simulink model "DCE_motor6_V2"  (R2025a)
settings: Solver=ode4  StartTime=0.0  StopTime=1  FixedStep=5e-5  RelTol=1e-3
undefined symbols (not defined in the file or in its folder): powergui
libraries: spsControlledVoltageSourceLib x24, spsControlledCurrentSourceLib x24, spsVoltageMeasurementLib x24, slpidlib x24, spspowerguiLib x2, simulink x1
(part 1 of 5)
settings Model: Creator=One  LastModifiedBy=One

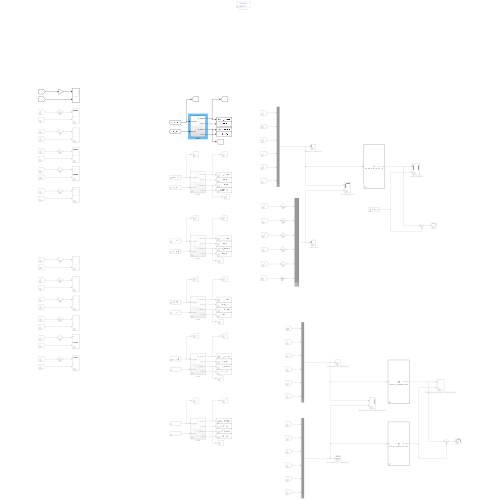
[thumbnail: Simulink's stored preview of the top-level diagram]
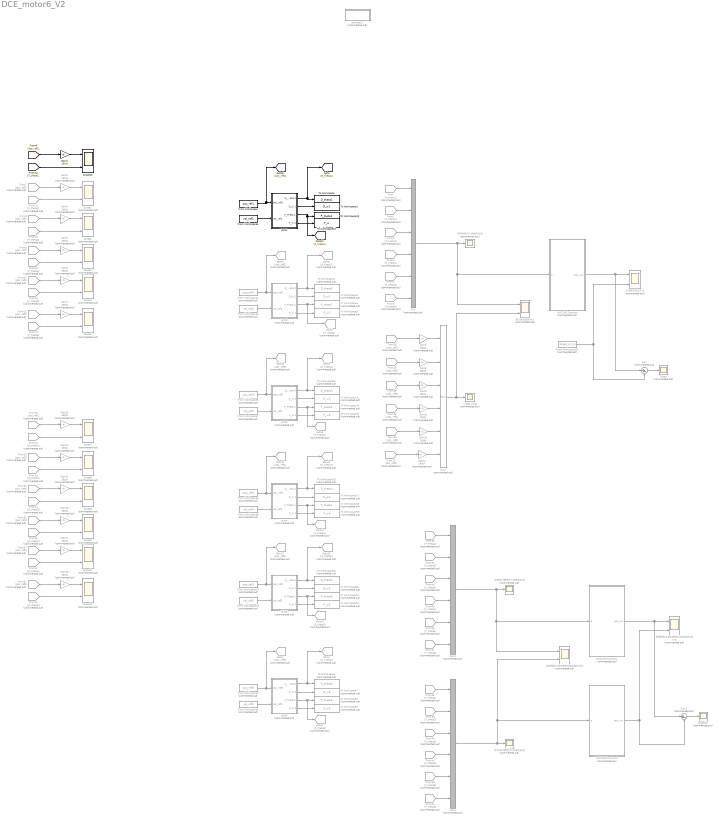
== system DCE_motor6_V2 ==
  From : From  Commented=on  GotoTag=P_theta1
  From Workspace : FromWorkspace  VariableName=pos_ref1
  From Workspace1 : FromWorkspace  VariableName=vel_ref1
  From Workspace10 : FromWorkspace  Commented=on  VariableName=pos_ref5
  From Workspace11 : FromWorkspace  Commented=on  VariableName=vel_ref5
  From Workspace12 : FromWorkspace  Commented=on  VariableName=target_xyz_ts
  From Workspace2 : FromWorkspace  Commented=on  VariableName=pos_ref2
  From Workspace3 : FromWorkspace  Commented=on  VariableName=vel_ref2
  From Workspace4 : FromWorkspace  Commented=on  VariableName=pos_ref6
  From Workspace5 : FromWorkspace  Commented=on  VariableName=vel_ref6
  From Workspace6 : FromWorkspace  Commented=on  VariableName=pos_ref3
  From Workspace7 : FromWorkspace  Commented=on  VariableName=vel_ref3
  From Workspace8 : FromWorkspace  Commented=on  VariableName=pos_ref4
  From Workspace9 : FromWorkspace  Commented=on  VariableName=vel_ref4
  From{1,13,37,39} (4 alike) : From  Commented=on  GotoTag=P_theta2
  From10 : From  Commented=on  GotoTag=pos_ref5
  From11 : From  Commented=on  GotoTag=pos_ref6
  From{2,14,40..41} (4 alike) : From  Commented=on  GotoTag=P_theta3
  From{3,15,42,45} (4 alike) : From  Commented=on  GotoTag=P_theta4
  From{4,16,43,46} (4 alike) : From  Commented=on  GotoTag=P_theta5
  From{5,17,44,47} (4 alike) : From  Commented=on  GotoTag=P_theta6
  From18 : From  Commented=on  GotoTag=pos_ref5
  From19 : From  Commented=on  GotoTag=pos_ref6
  From20 : From  Commented=on  GotoTag=pos_ref5
  From21 : From  Commented=on  GotoTag=pos_ref6
  From22 : From  Commented=on  GotoTag=D_theta1
  From23 : From  Commented=on  GotoTag=D_theta2
  From24 : From  Commented=on  GotoTag=D_theta3
  From25 : From  Commented=on  GotoTag=D_theta4
  From26 : From  Commented=on  GotoTag=pos_ref1
  From27 : From  Commented=on  GotoTag=pos_ref2
  From28 : From  Commented=on  GotoTag=pos_ref3
  From29 : From  Commented=on  GotoTag=pos_ref4
  From30 : From  Commented=on  GotoTag=D_theta5
  From31 : From  Commented=on  GotoTag=D_theta6
  From32 : From  Commented=on  GotoTag=pos_ref1
  From33 : From  Commented=on  GotoTag=pos_ref2
  From34 : From  Commented=on  GotoTag=pos_ref3
  From35 : From  Commented=on  GotoTag=pos_ref4
  From36 : From  Commented=on  GotoTag=P_theta1
  From38 : From  Commented=on  GotoTag=P_theta1
  From7 : From  Commented=on  GotoTag=pos_ref2
  From8 : From  Commented=on  GotoTag=pos_ref3
  From9 : From  Commented=on  GotoTag=pos_ref4
  Gain1 : Gain  Gain=180/pi
  Gain{2..18} (17 alike) : Gain  Commented=on  Gain=180/pi
  Goto1 : Goto  Commented=on  GotoTag=D_theta2
  Goto10 : Goto  Commented=on  GotoTag=pos_ref3
  Goto11 : Goto  Commented=on  GotoTag=D_theta4
  Goto13 : Goto  Commented=on  GotoTag=P_theta4
  Goto14 : Goto  Commented=on  GotoTag=pos_ref4
  Goto15 : Goto  Commented=on  GotoTag=D_theta5
  Goto16 : Goto  Commented=on  GotoTag=P_theta5
  Goto17 : Goto  Commented=on  GotoTag=pos_ref5
  Goto2 : Goto  Commented=on  GotoTag=P_theta2
  Goto3 : Goto  Commented=on  GotoTag=pos_ref2
  Goto4 : Goto  Commented=on  GotoTag=D_theta6
  Goto5 : Goto  Commented=on  GotoTag=P_theta6
  Goto7 : Goto  Commented=on  GotoTag=pos_ref6
  Goto8 : Goto  Commented=on  GotoTag=D_theta3
  Goto9 : Goto  Commented=on  GotoTag=P_theta3
  MATLAB Function : MATLAB Function  Commented=on  TreatAsAtomicUnit=on
  MATLAB Function1 : MATLAB Function  Commented=on  TreatAsAtomicUnit=on
  MATLAB Function2 : MATLAB Function  Commented=on  TreatAsAtomicUnit=on
  Mux{,1..3} (4 alike) : Mux  Commented=on  Inputs=6
  Scope : Scope  Commented=on
      settings: ActiveDisplayYMinimum=-0.000289462730006549  ActiveDisplayYMaximum=0.00023302341865344758  DataLoggingVariableName=ScopeData23
  Scope{1..9,11..12} (11 alike) : Scope  Commented=on  NumInputPorts=2
      Scope1 settings: ActiveDisplayYMinimum=-6.0139753089882335  ActiveDisplayYMaximum=54.125777780894119  DataLoggingVariableName=ScopeData10
      Scope11 settings: ActiveDisplayYMinimum=-48.669169301784144  ActiveDisplayYMaximum=5.4076854779760151
      Scope12 settings: ActiveDisplayYMinimum=-67.194027910067419  ActiveDisplayYMaximum=7.4660031011186
      Scope2 settings: ActiveDisplayYMinimum=-1.7922912289033655  ActiveDisplayYMaximum=12.011135261509935  DataLoggingVariableName=ScopeData16
      Scope3 settings: ActiveDisplayYMinimum=-8.3713341887105024  ActiveDisplayYMaximum=75.342007698394539  DataLoggingVariableName=ScopeData17
      Scope4 settings: ActiveDisplayYMinimum=-48.669169301784144  ActiveDisplayYMaximum=5.4076854779760151  DataLoggingVariableName=ScopeData18
      Scope5 settings: ActiveDisplayYMinimum=-67.194027910067419  ActiveDisplayYMaximum=7.4660031011186  DataLoggingVariableName=ScopeData19
      Scope6 settings: ActiveDisplayYMinimum=-6.0139753089882335  ActiveDisplayYMaximum=54.125777780894119  DataLoggingVariableName=ScopeData2
      Scope7 settings: ActiveDisplayYMinimum=43.128388243187558  ActiveDisplayYMaximum=44.899957966289  DataLoggingVariableName=ScopeData3
      Scope8 settings: ActiveDisplayYMinimum=-1.7922912289033655  ActiveDisplayYMaximum=12.011135261509935  DataLoggingVariableName=ScopeData4
      Scope9 settings: ActiveDisplayYMinimum=-8.3713341887105024  ActiveDisplayYMaximum=75.342007698394539  DataLoggingVariableName=ScopeData6
  Scope10 : Scope  NumInputPorts=2
      settings: ActiveDisplayYMinimum=-5.5836965217991938  ActiveDisplayYMaximum=7.5409112355633887  DataLoggingVariableName=ScopeData24
  Scope13 : Scope  Commented=on
      settings: ActiveDisplayYMinimum=-0.000289462730006549  ActiveDisplayYMaximum=0.00023302341865344758  DataLoggingVariableName=ScopeData7
  Sum : Sum  Commented=on  Inputs=|+-
  Sum1 : Sum  Commented=on  Inputs=|+-
  To Workspace : ToWorkspace  VariableName=D_theta1  SaveFormat=Timeseries  SampleTime=-1
  To Workspace1 : ToWorkspace  VariableName=D_w1  SaveFormat=Timeseries  SampleTime=-1
  To Workspace10 : ToWorkspace  Commented=on  VariableName=D_theta3  SaveFormat=Timeseries  SampleTime=-1
  To Workspace11 : ToWorkspace  Commented=on  VariableName=D_w3  SaveFormat=Timeseries  SampleTime=-1
  To Workspace12 : ToWorkspace  VariableName=P_theta1  SaveFormat=Timeseries  SampleTime=-1
  To Workspace13 : ToWorkspace  VariableName=P_w  SaveFormat=Timeseries  SampleTime=-1
  To Workspace14 : ToWorkspace  Commented=on  VariableName=P_theta3  SaveFormat=Timeseries  SampleTime=-1
  To Workspace15 : ToWorkspace  Commented=on  VariableName=P_w3  SaveFormat=Timeseries  SampleTime=-1
  To Workspace16 : ToWorkspace  Commented=on  VariableName=D_theta4  SaveFormat=Timeseries  SampleTime=-1
  To Workspace17 : ToWorkspace  Commented=on  VariableName=D_w4  SaveFormat=Timeseries  SampleTime=-1
  To Workspace18 : ToWorkspace  Commented=on  VariableName=P_theta4  SaveFormat=Timeseries  SampleTime=-1
  To Workspace19 : ToWorkspace  Commented=on  VariableName=P_w4  SaveFormat=Timeseries  SampleTime=-1
  To Workspace2 : ToWorkspace  Commented=on  VariableName=D_theta2  SaveFormat=Timeseries  SampleTime=-1
  To Workspace20 : ToWorkspace  Commented=on  VariableName=D_theta5  SaveFormat=Timeseries  SampleTime=-1
  To Workspace21 : ToWorkspace  Commented=on  VariableName=D_w5  SaveFormat=Timeseries  SampleTime=-1
  To Workspace22 : ToWorkspace  Commented=on  VariableName=P_theta5  SaveFormat=Timeseries  SampleTime=-1
  To Workspace23 : ToWorkspace  Commented=on  VariableName=P_w5  SaveFormat=Timeseries  SampleTime=-1
  To Workspace3 : ToWorkspace  Commented=on  VariableName=D_w2  SaveFormat=Timeseries  SampleTime=-1
  To Workspace4 : ToWorkspace  Commented=on  VariableName=P_theta2  SaveFormat=Timeseries  SampleTime=-1
  To Workspace5 : ToWorkspace  Commented=on  VariableName=P_w2  SaveFormat=Timeseries  SampleTime=-1
  To Workspace6 : ToWorkspace  Commented=on  VariableName=D_theta6  SaveFormat=Timeseries  SampleTime=-1
  To Workspace7 : ToWorkspace  Commented=on  VariableName=D_w6  SaveFormat=Timeseries  SampleTime=-1
  To Workspace8 : ToWorkspace  Commented=on  VariableName=P_theta6  SaveFormat=Timeseries  SampleTime=-1
  To Workspace9 : ToWorkspace  Commented=on  VariableName=P_w6  SaveFormat=Timeseries  SampleTime=-1
  joint1 : Subsystem
  joint2 : Subsystem  Commented=on
  joint3 : Subsystem  Commented=on
  joint4 : Subsystem  Commented=on
  joint5 : Subsystem  Commented=on
  joint6 : Subsystem  Commented=on
  powergui1 : Subsystem  Commented=on  AncestorBlock=spspowerguiLib/powergui  InitFcn=powergui( 'InitFcn_Callback' , gcb , 0 , [ ] );  mask(PSB option menu block){SimulationMode=Discrete, SampleTime=5e-5, frequency=60, Iterations=50, frequencyindice=0, Pbase=100e6, ErrMax=1e-4, UnitsV=kV, UnitsW=MW, buscounter=0, FunctionMessages=off, echomessages=off, EnableUseOfTLC=off, CurrentSourceSwitches=off, DisableSnubberDevices=off, DisableRonSwitches=off, DisableVfSwitches=off, DisplayEquations=off, AutomaticDiscreteSolvers=off, SolverType=Tustin/Backward Euler (TBE), Interpol=off, ExternalGateDelay=off, methode=off, Ts=0, x0status=blocks, SPID=off, SwTol=0, HookPort=off, NonlinearTolerance=1e-4, nMaxIteration=100, ContinueOnMaxIteration=off, RestoreLinks=warning, ResistiveCurrentMeasurement=off, Frange=[0:2:500], Ylog=off, Xlog=on, ShowGrid=off, save=off, variable=ZData, structure=0, ZoomFFT=on, StartTime=0.0, cycles=1, DisplayStyle=1, fundamental=60, FreqAxis=off, MaxFrequency=1000, frequencyindicesteady=1, RmsSteady=1, display=off}
      mask prompts: SimulationMode "Simulation type:"; SampleTime "Sample time (s):"; frequency "Frequency (Hz):"; Iterations "Max iterations"; frequencyindice "Frequency (Hz)"; Pbase "Base power (VA)"; ErrMax "PQ tolerance (pu)"; UnitsV "Voltage units"; UnitsW "Power units"; buscounter "Load flow bus counter"; FunctionMessages "Disable Specialized Power Systems warnings"; echomessages "Display Specialized Power Systems compilation messages"; EnableUseOfTLC "Use TLC file when in Accelerator Simulation Mode and for code generation"; CurrentSourceSwitches "Disable ideal switching"; DisableSnubberDevices "Disable snubbers in switching devices"; DisableRonSwitches "Disable Ron resistances in switching devices"; DisableVfSwitches "Disable forward voltages in switching devices"; DisplayEquations "Display circuit differential equations"; AutomaticDiscreteSolvers "Automatically handle Discrete solver and Advanced tab solver settings of blocks"; SolverType "Discrete solver"; Interpol "Interpolate switching events"; ExternalGateDelay "Use time-stamped gate signals"; methode "Store switching topologies"; Ts "Buffer size (MBytes):"; x0status "Start simulation with initial electrical states from:"; SPID "Use ideal switching devices"; SwTol "Switch tolerance"; HookPort "Allow multiple powergui blocks"; NonlinearTolerance "Solver tolerance"; nMaxIteration "Maximum number of iterations"; ContinueOnMaxIteration "Continue Simulation if maximum number of iterations is reached"; RestoreLinks "Restore disabled links of Simscape Power Systems ST blocks:"; ResistiveCurrentMeasurement "Use non ideal current measurement blocks (1e-4Ohm internal resistance)"; Frange "Frequency Range"; Ylog "Log impedance"; Xlog "log Frequency"; ShowGrid "grid"; save "Save Data To Workspace"; variable "Variable Name"; structure "Structure Name (PSBFFTSCOPE)"; ZoomFFT "ZoomFFT (PSBFFTSCOPE)"; StartTime "Start Time (PSBFFTSCOPE)"; cycles "Cycles (PSBFFTSCOPE)"; DisplayStyle "Display style (PSBFFTSCOPE)"; fundamental "Fundamental (PSBFFTSCOPE)"; FreqAxis "Frequency Axis (PSBFFTSCOPE)"; MaxFrequency "Max Frequency (PSBFFTSCOPE)"; frequencyindicesteady "Frequency indice (STEADYSTATE)"; RmsSteady "RMS display (STEADYSTATE)"; display "Display Results"
      mask help: Set simulation type, simulation parameters, and preferences.
      mask init:
      | dispMessage = '';
      | dispMessage = powergui('MaskInitialization',gcb,SimulationMode,SampleTime);
      settings: PreSaveFcn=powergui( 'PreSaveFcn_Callback' , gcb , [ ] , [ ] );  OpenFcn=sps_rtmsupport('OpenFcn',gcbh)
      mask Help: helpview(psbhelp)
      mask TypeOptions SimulationMode: Continuous | Discrete | Phasor | Discrete phasor
      mask Callback SimulationMode: powergui('SimulationType',[],[],gcb);
      mask TypeOptions UnitsV: V | kV
      mask TypeOptions UnitsW: W | kW | MW
      mask Callback CurrentSourceSwitches: powergui('SimulationType',[],[],gcb);
      mask Callback AutomaticDiscreteSolvers: powergui('SimulationType',[],[],gcb);
      mask TypeOptions SolverType: Tustin/Backward Euler (TBE) | Tustin | Backward Euler
      mask Callback SolverType: powergui('SimulationType',[],[],gcb);
      mask Callback Interpol: powergui('SimulationType',[],[],gcb);
      mask Callback ExternalGateDelay: powergui('SimulationType',[],[],gcb);
      mask Callback methode: powergui('SimulationType',[],[],gcb);
      mask TypeOptions x0status: blocks | steady | zero
      mask TypeOptions RestoreLinks: yes | warning | no
      mask Callback display: sps_rtmsupport('parametereditingmodes',gcbh) % Will be executed last in parameter callbacks to ensure mask enable consistency
      mask DialogControl SolverTab Prompt: Solver
      mask DialogControl AutoSolverNote Prompt: The Simulation type parameter is governed by Simulink. To access the Powergui solver settings, unselect auto (Automatic solver selection) solver in the Simulink solver options.
      mask DialogControl Apps Prompt: Apps
      mask DialogControl StateAnalyzer Prompt: Measurements and States Analyzer
      mask DialogControl StateAnalyzer Callback: powerStates(bdroot(gcb))
      mask DialogControl LineParameterCalculator Prompt: Line Parameter Calculator
      mask DialogControl LineParameterCalculator Callback:
      | close_system(gcb)
      | powerLineParameters
      mask DialogControl CableParameterCalculator Prompt: Cable Parameter Calculator
      mask DialogControl CableParameterCalculator Callback:
      | close_system(gcb)
      | powerCableParameters
      mask DialogControl LineDecoupler Prompt: Line Decoupler
      mask DialogControl LineDecoupler Tooltip: Click to replace selected Distributed Parameters Line blocks with Decoupling Line blocks
      mask DialogControl LineDecoupler Callback:
      | close_system(gcb);
      | DecouplingLineReplace(gcs)
      mask DialogControl LoadFlowAnalyzer Prompt: Load Flow Analyzer
      mask DialogControl LoadFlowAnalyzer Callback:
      | close_system(gcb)
      | powerLoadFlow
      mask DialogControl LoadFlowParameters Prompt: Load Flow Parameters
      mask DialogControl ImpedanceCalculator Prompt: Impedance Calculator
      mask DialogControl ImpedanceCalculator Callback:
      | close_system(gcb);
      | powerImpedance(bdroot(gcs));
      mask DialogControl FFTAnalyzer Prompt: FFT Analyzer
      mask DialogControl FFTAnalyzer Callback:
      | close_system(gcb)
      | power_fftscope(bdroot(gcb),gcb)
      mask DialogControl LinearSystemAnalyzer Prompt: Linear System Analyzer
      mask DialogControl LinearSystemAnalyzer Callback:
      | close_system(gcb)
      | power_ltiview(bdroot(gcb))
      mask DialogControl HysteresisDesigner Prompt: Hysteresis Designer
      mask DialogControl HysteresisDesigner Callback:
      | close_system(gcb)
      | powerHysteresis('hysteresis.mat')
      mask DialogControl BlockCustomizer Prompt: Block Customizer
      mask DialogControl BlockCustomizer Callback:
      | close_system(gcb);
      | power_customize;
      mask DialogControl ReportGenerator Prompt: Report Generator
      mask DialogControl ReportGenerator Callback:
      | close_system(gcb)
      | power_report(bdroot(gcb))
      mask DialogControl obsolete Prompt: ...
      mask DialogControl MachineInitialization Prompt: Machine Initialization
      mask DialogControl MachineInitialization Callback:
      | close_system(gcb)
      | powericon('machineInitTool',bdroot(gcb),gcb)
      mask DialogControl Preferences Prompt: Preferences
      mask DialogControl Solver Prompt: Solver
      mask DialogControl SolverDetails Prompt: Solver details for nonlinear elements
      mask Display: color('blue'),disp(dispMessage)
  六条输入轨迹 : Scope  Commented=on
      settings: DataLoggingVariableName=ScopeData20
  实物电机模型的六条输出轨迹 : Scope  Commented=on
      settings: ActiveDisplayYMinimum=-75.563478283435458  ActiveDisplayYMaximum=82.802808576726292  DataLoggingVariableName=ScopeData9
  实物电机的六条输出轨迹 : Scope  Commented=on
      settings: ActiveDisplayYMinimum=-75.563478283435458  ActiveDisplayYMaximum=82.802808576726292  DataLoggingVariableName=ScopeData15
  尖端电机轨迹XYZ : Scope  Commented=on  NumInputPorts=2
      settings: ActiveDisplayYMinimum=-0.074441825005112566  ActiveDisplayYMaximum=0.66483489550037078  DataLoggingVariableName=ScopeData22
  数字电机模型的六条输出轨迹 : Scope  Commented=on
      settings: DataLoggingVariableName=ScopeData8
  物理模型与数字模型的尖端电机轨迹XYZ : Scope  Commented=on  NumInputPorts=2
      settings: ActiveDisplayYMinimum=-0.061507125001366951  ActiveDisplayYMaximum=0.37025412500015187  DataLoggingVariableName=ScopeData11
  物理模型与数字模型的输出曲线对比 : Scope  Commented=on  NumInputPorts=2
      settings: ActiveDisplayYMinimum=-75.563478283435458  ActiveDisplayYMaximum=82.802808576726292  DataLoggingVariableName=ScopeData12
  输入输出曲线对比 : Scope  Commented=on  NumInputPorts=2
      settings: ActiveDisplayYMinimum=-75.563478283435458  ActiveDisplayYMaximum=82.802808576726292  DataLoggingVariableName=ScopeData21
  wires:
  From/1 -> Mux/1
  From1/1 -> Mux/2
  From2/1 -> Mux/3
  From3/1 -> Mux/4
  From4/1 -> Mux/5
  From5/1 -> Mux/6
  Mux/1 -> MATLAB Function/1(q), 输入输出曲线对比/1, 实物电机的六条输出轨迹/1
  [pos_ref1] -> Gain1/1
  From7/1 -> Gain2/1
  From8/1 -> Gain4/1
  From9/1 -> Gain5/1
  From10/1 -> Gain6/1
  From11/1 -> Gain7/1
  Gain1/1 -> Scope10/1
  Gain2/1 -> Scope1/1
  Gain4/1 -> Scope2/1
  Gain5/1 -> Scope3/1
  Gain6/1 -> Scope4/1
  Gain7/1 -> Scope5/1
  [P_theta1] -> Scope10/2
  From13/1 -> Scope1/2
  From14/1 -> Scope2/2
  From15/1 -> Scope3/2
  From16/1 -> Scope4/2
  From17/1 -> Scope5/2
  From26/1 -> Gain3/1
  From27/1 -> Gain8/1
  Gain3/1 -> Mux1/1
  From28/1 -> Gain9/1
  From29/1 -> Gain10/1
  Gain11/1 -> Mux1/5
  From19/1 -> Gain12/1
  Gain10/1 -> Mux1/4
  Gain12/1 -> Mux1/6
  Gain8/1 -> Mux1/2
  From18/1 -> Gain11/1
  Gain9/1 -> Mux1/3
  Mux1/1 -> 输入输出曲线对比/2, 六条输入轨迹/1
  MATLAB Function/1(pos_xyz) -> Sum/1, 尖端电机轨迹XYZ/1
  From Workspace12/1 -> Sum/2, 尖端电机轨迹XYZ/2
  Sum/1 -> Scope/1
  From Workspace/1 -> [pos_ref1], joint1/1(pos_ref1)
  From Workspace1/1 -> joint1/2(vel_ref1)
  joint1/1(D_Theta 1) -> To Workspace/1, [D_theta1]
  joint1/2(D_w 1) -> To Workspace1/1
  joint1/3(P_Theta 1) -> [P_theta1], To Workspace12/1
  joint1/4(P_w 1) -> To Workspace13/1
  From Workspace3/1 -> joint2/2(vel_ref2)
  joint2/2(D_w 2) -> To Workspace3/1
  joint2/3(P_Theta 2) -> Goto2/1, To Workspace4/1
  joint2/4(P_w 2) -> To Workspace5/1
  joint2/1(D_Theta 2) -> To Workspace2/1, Goto1/1
  From Workspace2/1 -> Goto3/1, joint2/1(pos_ref2)
  From Workspace7/1 -> joint3/2(vel_ref3)
  joint3/2(D_w 3) -> To Workspace11/1
  joint3/3(P_Theta 3) -> Goto9/1, To Workspace14/1
  joint3/4(P_w 3) -> To Workspace15/1
  joint3/1(D_Theta 3) -> To Workspace10/1, Goto8/1
  From Workspace6/1 -> Goto10/1, joint3/1(pos_ref3)
  From Workspace9/1 -> joint4/2(vel_ref4)
  joint4/2(D_w 4) -> To Workspace17/1
  joint4/3(P_Theta 4) -> Goto13/1, To Workspace18/1
  joint4/4(P_w 4) -> To Workspace19/1
  joint4/1(D_Theta 4) -> To Workspace16/1, Goto11/1
  From Workspace8/1 -> Goto14/1, joint4/1(pos_ref4)
  From Workspace11/1 -> joint5/2(vel_ref5)
  joint5/2(D_w 5) -> To Workspace21/1
  joint5/3(P_Theta 5) -> Goto16/1, To Workspace22/1
  joint5/4(P_w 5) -> To Workspace23/1
  joint5/1(D_Theta 5) -> To Workspace20/1, Goto15/1
  From Workspace10/1 -> Goto17/1, joint5/1(pos_ref5)
  joint6/1(D_Theta 6) -> To Workspace6/1, Goto4/1
  joint6/2(D_w 6) -> To Workspace7/1
  joint6/4(P_w 6) -> To Workspace9/1
  joint6/3(P_Theta 6) -> Goto5/1, To Workspace8/1
  From Workspace5/1 -> joint6/2(vel_ref6)
  From Workspace4/1 -> Goto7/1, joint6/1(pos_ref6)
  From30/1 -> Scope11/2
  From25/1 -> Scope9/2
  From22/1 -> Scope7/2
  Gain17/1 -> Scope11/1
  From23/1 -> Scope6/2
  From24/1 -> Scope8/2
  Gain15/1 -> Scope8/1
  From31/1 -> Scope12/2
  Gain14/1 -> Scope6/1
  From33/1 -> Gain14/1
  Gain16/1 -> Scope9/1
  From32/1 -> Gain13/1
  Gain18/1 -> Scope12/1
  From20/1 -> Gain17/1
  From21/1 -> Gain18/1
  From34/1 -> Gain15/1
  From35/1 -> Gain16/1
  Gain13/1 -> Scope7/1
  From37/1 -> Mux2/2
  From47/1 -> Mux2/6
  MATLAB Function1/1(pos_xyz) -> Sum1/1, 物理模型与数字模型的尖端电机轨迹XYZ/1
  From46/1 -> Mux2/5
  From36/1 -> Mux2/1
  Sum1/1 -> Scope13/1
  From40/1 -> Mux2/3
  From45/1 -> Mux2/4
  Mux2/1 -> MATLAB Function1/1(q), 物理模型与数字模型的输出曲线对比/1, 实物电机模型的六条输出轨迹/1
  Mux3/1 -> 物理模型与数字模型的输出曲线对比/2, MATLAB Function2/1(q), 数字电机模型的六条输出轨迹/1
  From42/1 -> Mux3/4
  From41/1 -> Mux3/3
  From38/1 -> Mux3/1
  From44/1 -> Mux3/6
  From43/1 -> Mux3/5
  From39/1 -> Mux3/2
  MATLAB Function2/1(pos_xyz) -> Sum1/2, 物理模型与数字模型的尖端电机轨迹XYZ/2

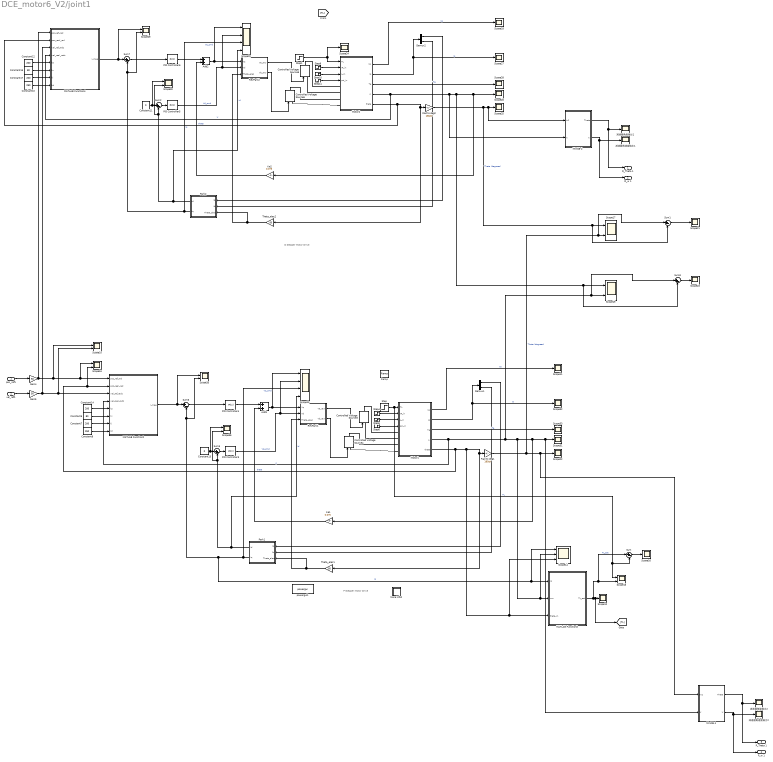
== system DCE_motor6_V2/joint1 ==
  note: D Stepper Motor Drive
  note: P Stepper Motor Drive
  pos_ref1 : Inport
  vel_ref1 : Inport  Port=2
  Add1 : Sum
  Add2 : Sum
  Constant10 : Constant  Value=250
  Constant11 : Constant  Value=0
  Constant{7,12,14,17} (4 alike) : Constant  Value=200
  Constant13 : Constant  Value=0
  Constant15 : Constant  Value=80
  Constant6 : Constant  Value=80
  Constant8 : Constant  Value=250
  Controlled Voltage Source{3..6} (4 alike) : spsControlledVoltageSourceLib/Controlled Voltage Source  Initialize=on  Source_Type=AC  Amplitude=0  Phase=0  Frequency=0  Measurements=None
  Demux1 : Demux  Outputs=2
  Demux2 : Demux  Outputs=2
  Gain4 : Gain  Gain=50
  Gain5 : Gain  Gain=50
  Ke1 : Gain  Gain=0.075
  Ke2 : Gain  Gain=0.075
  MATLAB Function2 : MATLAB Function  TreatAsAtomicUnit=on
  MATLAB Function3 : MATLAB Function  TreatAsAtomicUnit=on
  MATLAB Function4 : MATLAB Function  TreatAsAtomicUnit=on
  Mini08-1 : Subsystem
  Mini08-2 : Subsystem
  More Info2 : Subsystem
      settings: OpenFcn="showExample(\"simscapeelectricalsps/StepperMotorExample\")"
      mask Display: disp('?')
  Motor1 : Subsystem
  Motor2 : Subsystem
  PID Controller{3..6} (4 alike) : slpidlib/PID Controller  Controller=PI  Form=Parallel  TimeDomain=Discrete-time  UseExternalTs=off  SampleTime=5e-5  IntegratorMethod=Forward Euler  FilterMethod=Forward Euler  ControllerParametersSource=internal  P=5  I=4000  UseKiTs=off  D=0  UseExternalDerivativeSource=off  N=100  UseFilter=on  TunerSelectOption=Transfer Function Based (PID Tuner App)  InitialConditionSource=internal  InitialConditionForIntegrator=0  InitialConditionForFilter=0  DifferentiatorICPrevScaledInput=0  ExternalReset=none  TrackingMode=off  Kt=1  LimitOutput=on  SatLimitsSource=internal  UpperSaturationLimit=24  LowerSaturationLimit=-24  LinearizeAsGain=on  AntiWindupMode=clamping  Kb=1  LimitIntegrator=on  UpperIntegratorSaturationLimit=24  LowerIntegratorSaturationLimit=-24  POutMin=[]  POutMax=[]  IOutMin=[]  IOutMax=[]  DOutMin=[]  DOutMax=[]  NOutMin=[]  NOutMax=[]  SumOutMin=[]  SumOutMax=[]  SaturationOutMin=[]  SaturationOutMax=[]  PParamMin=[]  PParamMax=[]  IParamMin=[]  IParamMax=[]  DParamMin=[]  DParamMax=[]  NParamMin=[]  NParamMax=[]  KbParamMin=[]  KbParamMax=[]  KtParamMin=[]  KtParamMax=[]  KbOutMin=[]  KbOutMax=[]  KtOutMin=[]  KtOutMax=[]  IntegratorOutMin=[]  IntegratorOutMax=[]  FilterOutMin=[]  FilterOutMax=[]  SumI1OutMin=[]  SumI1OutMax=[]  SumI2OutMin=[]  SumI2OutMax=[]  SumI3OutMin=[]  SumI3OutMax=[]  SumI4OutMin=[]  SumI4OutMax=[]  SumDOutMin=[]  SumDOutMax=[]  DifferentiatorOutMin=[]  DifferentiatorOutMax=[]  FilterDiffOutCoefMin=[]  FilterDiffOutCoefMax=[]  ReciprocalOutMin=[]  ReciprocalOutMax=[]  SumDenOutMin=[]  SumDenOutMax=[]  SumNumOutMin=[]  SumNumOutMax=[]  DivideOutMin=[]  DivideOutMax=[]  UdiffTsProdOutMin=[]  UdiffTsProdOutMax=[]  NTsProdOutMin=[]  NTsProdOutMax=[]  UintegralTsProdOutMin=[]  UintegralTsProdOutMax=[]  UngainTsProdOutMin=[]  UngainTsProdOutMax=[]  ClampingZeroOutDataTypeStr=Inherit: Inherit via back propagation  ClampingZeroOutMin=[]  ClampingZeroOutMax=[]  FilterDenConstantOutDataTypeStr=Inherit: Inherit via back propagation  FilterDenConstantOutMin=[]  FilterDenConstantOutMax=[]  PCopyOutDataTypeStr=Inherit: Inherit via back propagation  PCopyOutMin=[]  PCopyOutMax=[]  NCopyOutDataTypeStr=Inherit: Inherit via back propagation  NCopyOutMin=[]  NCopyOutMax=[]  IntegratorContinuousStateAttributes=''  IntegratorStateMustResolveToSignalObject=off  IntegratorRTWStateStorageClass=Auto  FilterContinuousStateAttributes=''  FilterStateMustResolveToSignalObject=off  FilterRTWStateStorageClass=Auto  ParallelPVariant=InternalParameters  IdealPVariant=Disabled  IVariant=InternalParameters  DVariant=Disabled  IntegratorVariant=Discrete  SatVariant=Enabled  AWVariant=DiscClampingParallel  PCopyVariant=Disabled  TRVariant=Disabled  FdbkBlocksVariant=Forward  IdealPFdbkVariant=Disabled  SatFdbkVariant=Disabled  DerivativeFilterVariant=Disabled  NVariant=Disabled  NCopyVariant=Disabled_SignalSpec  FilterICVariant=Disabled  IntegratorICVariant=InternalICs  ExternalResetVariant=Disabled  TRSumVariant=Passthrough  SumFdbkVariant=Disabled  SumVariant=Sum_PI  TsampFilterVariant=InternalTs  TsampNgainVariant=Passthrough  TsampIntegralVariant=Disabled_SignalSpec  ExternalSaturationOutDataTypeStr=Inherit: Same as second input  DerivativeSourceVariant=Disabled  PreIntVariant=InternalPreInt
  Park1 : MATLAB Function  TreatAsAtomicUnit=on
  Park2 : MATLAB Function  TreatAsAtomicUnit=on
  Rad to deg1 : Gain  Gain=180/pi
  Rad to deg2 : Gain  Gain=180/pi
  Ramp : simulink/Sources/Ramp  slope=0.006  start=0  InitialOutput=0.01
  RevPark1 : MATLAB Function  TreatAsAtomicUnit=on
  RevPark2 : MATLAB Function  TreatAsAtomicUnit=on
  Scope{10,15,17,19,29..30,34..36} (9 alike) : Scope  NumInputPorts=2
      Scope10 settings: ActiveDisplayYMinimum=-5.2481835137744008  ActiveDisplayYMaximum=47.233651623969614  DataLoggingVariableName=ScopeData27
      Scope15 settings: ActiveDisplayYMinimum=0.00625  ActiveDisplayYMaximum=0.04375  DataLoggingVariableName=ScopeData34
      Scope17 settings: ActiveDisplayYMinimum=-287.89976310434338  ActiveDisplayYMaximum=575.16137858375225  DataLoggingVariableName=ScopeData36
      Scope19 settings: ActiveDisplayYMinimum=-24.982969715205265  ActiveDisplayYMaximum=69.499857868635672  DataLoggingVariableName=ScopeData38
      Scope29 settings: ActiveDisplayYMinimum=-0.018504547079538081  ActiveDisplayYMaximum=0.49853620070628168  DataLoggingVariableName=ScopeData28
      Scope30 settings: ActiveDisplayYMinimum=-0.068250226127922337  ActiveDisplayYMaximum=0.064256506451961737  DataLoggingVariableName=ScopeData29
      Scope34 settings: ActiveDisplayYMinimum=37.665150555747651  ActiveDisplayYMaximum=39.407336225091846  DataLoggingVariableName=ScopeData49
      Scope35 settings: ActiveDisplayYMinimum=-0.018504547079538081  ActiveDisplayYMaximum=0.49853620070628168  DataLoggingVariableName=ScopeData50
      Scope36 settings: ActiveDisplayYMinimum=-0.068250226127922337  ActiveDisplayYMaximum=0.064256506451961737  DataLoggingVariableName=ScopeData51
  Scope{11..12,16,18,21..28,31..33} (15 alike) : Scope
      Scope11 settings: ActiveDisplayYMinimum=-19.096901402816375  ActiveDisplayYMaximum=19.120590576315788  DataLoggingVariableName=ScopeData30
      Scope12 settings: ActiveDisplayYMinimum=-0.005028035303192257  ActiveDisplayYMaximum=0.045252317728730319  DataLoggingVariableName=ScopeData31
      Scope16 settings: ActiveDisplayYMinimum=-0.00045623090907525666  ActiveDisplayYMaximum=0.00044225246132360179  DataLoggingVariableName=ScopeData35
      Scope18 settings: ActiveDisplayYMinimum=-19.096901402816375  ActiveDisplayYMaximum=19.120590576315788  DataLoggingVariableName=ScopeData37
      Scope21 settings: ActiveDisplayYMinimum=-6.1502055823969322  ActiveDisplayYMaximum=1.5579460890257923  DataLoggingVariableName=ScopeData40
      Scope22 settings: ActiveDisplayYMinimum=-1073.0161987450256  ActiveDisplayYMaximum=478.45817124156184  DataLoggingVariableName=ScopeData41
      Scope23 settings: ActiveDisplayYMinimum=-6.5852940186487112  ActiveDisplayYMaximum=6.2413973243820795  DataLoggingVariableName=ScopeData42
      Scope24 settings: ActiveDisplayYMinimum=-0.019291388561127311  ActiveDisplayYMaximum=0.055061528118044607  DataLoggingVariableName=ScopeData43
      Scope25 settings: ActiveDisplayYMinimum=-101.39982984513261  ActiveDisplayYMaximum=451.43127016035271  DataLoggingVariableName=ScopeData44
      Scope26 settings: ActiveDisplayYMinimum=-452.6835395386438  ActiveDisplayYMaximum=318.93705127381384  DataLoggingVariableName=ScopeData45
      Scope27 settings: ActiveDisplayYMinimum=-0.40449771436693455  ActiveDisplayYMaximum=0.64067173662257559  DataLoggingVariableName=ScopeData25
      Scope28 settings: ActiveDisplayYMinimum=-0.046646220623980633  ActiveDisplayYMaximum=0.10063848186154864  DataLoggingVariableName=ScopeData26
      Scope31 settings: ActiveDisplayYMinimum=-108.68072883446378  ActiveDisplayYMaximum=111.31923817185427  DataLoggingVariableName=ScopeData46
      Scope32 settings: ActiveDisplayYMinimum=-0.40449771436693455  ActiveDisplayYMaximum=0.64067173662257559  DataLoggingVariableName=ScopeData47
      Scope33 settings: ActiveDisplayYMinimum=-0.046646220623980633  ActiveDisplayYMaximum=0.10063848186154864  DataLoggingVariableName=ScopeData48
  Scope13 : Scope  NumInputPorts=4
      settings: ActiveDisplayYMinimum=-0.68813129304418319  ActiveDisplayYMaximum=6.2555990509558841  DataLoggingVariableName=ScopeData32
  Scope14 : Scope  NumInputPorts=3
      settings: ActiveDisplayYMinimum=-0.052783691584462819  ActiveDisplayYMaximum=0.4750532242601655  DataLoggingVariableName=ScopeData33
  Scope20 : Scope  NumInputPorts=4
      settings: ActiveDisplayYMinimum=-0.68813129304418319  ActiveDisplayYMaximum=6.2555990509558841  DataLoggingVariableName=ScopeData39
  Step : Step  Time=0.5  Before=0.005  After=0.04  SampleTime=0
  Step1 : Step  Time=0  Before=0.005  After=0.005  SampleTime=0
  Step10 : Step  Time=0  Before=0.00544  After=0.00544  SampleTime=0
  Step11 : Step  Time=0  Before=0.0015  After=0.0015  SampleTime=0
  Step4 : Step  Time=0  Before=4.85  After=4.85  SampleTime=0
  Step5 : Step  Time=0  Before=0.00544  After=0.00544  SampleTime=0
  Step6 : Step  Time=0  Before=0.0015  After=0.0015  SampleTime=0
  Step9 : Step  Time=0  Before=4.85  After=4.85  SampleTime=0
  Sum{,1..2,5..8} (7 alike) : Sum  Inputs=|+-
  Theta_elec1 : Gain  Gain=50
  Theta_elec2 : Gain  Gain=50
  powergui1 : spspowerguiLib/powergui  SimulationMode=Discrete  SampleTime=5e-5  frequency=60  Iterations=50  frequencyindice=0  Pbase=100e6  ErrMax=1e-4  UnitsV=kV  UnitsW=MW  buscounter=0  FunctionMessages=off  echomessages=off  EnableUseOfTLC=off  CurrentSourceSwitches=off  DisableSnubberDevices=off  DisableRonSwitches=off  DisableVfSwitches=off  DisplayEquations=off  AutomaticDiscreteSolvers=off  SolverType=Tustin/Backward Euler (TBE)  Interpol=off  ExternalGateDelay=off  methode=off  Ts=0  x0status=blocks  SPID=off  SwTol=0  HookPort=off  NonlinearTolerance=1e-4  nMaxIteration=100  ContinueOnMaxIteration=off  RestoreLinks=warning  ResistiveCurrentMeasurement=off  Frange=[0:2:500]  Ylog=off  Xlog=on  ShowGrid=off  save=off  variable=ZData  structure=0  ZoomFFT=on  StartTime=0.0  cycles=1  DisplayStyle=1  fundamental=60  FreqAxis=off  MaxFrequency=1000  frequencyindicesteady=1  RmsSteady=1  display=off
  减速器角度输出1 : Scope
      settings: ActiveDisplayYMinimum=-3.2575204385667078  ActiveDisplayYMaximum=25.318176358378867  DataLoggingVariableName=ScopeData53
  减速器角度输出2 : Scope
      settings: ActiveDisplayYMinimum=-3.2575204385667078  ActiveDisplayYMaximum=25.318176358378867  DataLoggingVariableName=ScopeData56
  减速器角速度输出1 : Scope
      settings: ActiveDisplayYMinimum=-0.049701649268213327  ActiveDisplayYMaximum=0.44324985732957672  DataLoggingVariableName=ScopeData54
  减速器角速度输出2 : Scope
      settings: ActiveDisplayYMinimum=-0.049701649268213327  ActiveDisplayYMaximum=0.44324985732957672  DataLoggingVariableName=ScopeData57
  D_Theta 1 : Outport
  D_w 1 : Outport  Port=2
  P_Theta 1 : Outport  Port=3
  P_w 1 : Outport  Port=4
  wires:
  Sum8/1 -> Scope23/1
  Sum1/1 -> Scope21/1
  Motor2/1(Vp) -> Scope18/1  "Vp"
  Motor2/2(Ip) -> Demux2/1, Scope27/1  "Ip"
  Park2/2(Iq) -> Scope20/3, Scope29/2, Sum7/2  "Iq"
  Park2/1(Id) -> Scope20/4, Scope30/2, Sum2/2  "Id"
  Constant11/1 -> Scope30/1, Sum2/1
  PID Controller6/1 -> Add2/1
  MATLAB Function4/1(I_mag) -> Scope29/1, Sum7/1
  Demux2/1 -> Park2/1(Ia)
  Sum7/1 -> PID Controller6/1
  Motor2/5(theta) -> MATLAB Function4/2(pos_real_rad), Rad to deg2/1, Theta_elec2/1  "theta"
  Constant12/1 -> MATLAB Function4/5(kp)
  Sum2/1 -> PID Controller5/1
  Step10/1 -> Motor2/3(L_in)
  Ke2/1 -> Add2/2
  Motor2/3(Te) -> Scope28/1  "Te"
  RevPark2/2(Vb_raw) -> Controlled Voltage Source6/1
  Step11/1 -> Motor2/4(psi_in)
  Theta_elec2/1 -> RevPark2/3(Theta_elec), Park2/3(Theta_elec)
  Constant17/1 -> MATLAB Function4/7(ki)
  Add2/1 -> Scope20/1, RevPark2/1(Vq)  "Vq_cmd"
  PID Controller5/1 -> Scope20/2, RevPark2/2(Vd)  "Vd_cmd"
  Step/1 -> Sum/2, Scope15/1, Motor1/1(TL)  "TL"
  Motor2/4(w) -> MATLAB Function4/4(vel_real_rads), Mini08-2/2(w), Sum8/2, Scope19/1, Ke2/1, Scope26/1  "w"
  MATLAB Function3/1(TL_est) -> Sum/1, Scope15/2, [TL], Scope12/1  "TL_est"
  Sum/1 -> Scope16/1
  PID Controller3/1 -> Scope13/2, RevPark1/2(Vd)  "Vd_cmd"
  Motor1/4(w) -> MATLAB Function2/4(vel_real_rads), Sum8/1, Scope19/2, Scope14/2, MATLAB Function3/2(wm), Ke1/1, Mini08-1/2(w), Scope31/1  "w"
  Step9/1 -> Motor2/2(IR_in)
  Add1/1 -> Scope13/1, RevPark1/1(Vq)  "Vq_cmd"
  Constant14/1 -> MATLAB Function2/5(kp)
  Park1/1(Id) -> Scope13/4, Scope36/2, Sum5/2  "Id"
  Constant6/1 -> MATLAB Function2/6(kv)
  Constant15/1 -> MATLAB Function4/6(kv)
  Constant7/1 -> MATLAB Function2/7(ki)
  Theta_elec1/1 -> RevPark1/3(Theta_elec), Park1/3(Theta_elec)
  Motor1/5(theta) -> Scope34/2, MATLAB Function2/2(pos_real_rad), Scope14/3, MATLAB Function3/3(theta_m), Rad to deg1/1, Theta_elec1/1  "theta"
  Sum5/1 -> PID Controller3/1
  Step5/1 -> Motor1/3(L_in)
  Ke1/1 -> Add1/2
  Step6/1 -> Motor1/4(psi_in)
  Sum6/1 -> PID Controller4/1
  Rad to deg1/1 -> Sum1/1, Scope17/2, Mini08-1/1(In2), Scope22/1  "Theta (degrees)"
  RevPark1/2(Vb_raw) -> Controlled Voltage Source4/1
  Demux2/2 -> Park2/2(Ib)
  Motor1/3(Te) -> Scope33/1  "Te"
  Rad to deg2/1 -> Sum1/2, Scope17/1, Mini08-2/1(In2), Scope25/1  "Theta (degrees)"
  RevPark1/1(Va_raw) -> Controlled Voltage Source3/1
  Constant8/1 -> MATLAB Function2/8(kd)
  Demux1/1 -> Park1/1(Ia)
  Motor1/1(Vp) -> Scope11/1  "Vp"
  RevPark2/1(Va_raw) -> Controlled Voltage Source5/1
  Step4/1 -> Motor1/2(IR_in)
  Park1/2(Iq) -> Scope13/3, Scope14/1, MATLAB Function3/1(iq), Scope35/2, Sum6/2  "Iq"
  Constant10/1 -> MATLAB Function4/8(kd)
  MATLAB Function2/1(I_mag) -> Scope35/1, Sum6/1
  Motor1/2(Ip) -> Demux1/1, Scope32/1  "Ip"
  Constant13/1 -> Scope36/1, Sum5/1
  PID Controller4/1 -> Add1/1
  Demux1/2 -> Park1/2(Ib)
  vel_ref1/1 -> Gain5/1
  Gain4/1 -> Scope10/1, Scope34/1, MATLAB Function2/1(pos_ref_rad), MATLAB Function4/1(pos_ref_rad)
  pos_ref1/1 -> Gain4/1
  Gain5/1 -> Scope10/2, MATLAB Function2/3(vel_ref_rads), MATLAB Function4/3(vel_ref_rads)
  Mini08-2/1("Theta ") -> D_Theta 1/1, 减速器角度输出1/1
  Mini08-2/2("w ") -> D_w 1/1, 减速器角速度输出1/1
  Mini08-1/2("w ") -> P_w 1/1, 减速器角速度输出2/1
  Mini08-1/1("Theta ") -> P_Theta 1/1, 减速器角度输出2/1
  Step1/1 -> Motor2/1(TL), Scope24/1
  connections:
  Motor1/LConn4 -- Controlled Voltage Source4/LConn1
  Motor2/LConn4 -- Controlled Voltage Source6/LConn1
  Motor1/LConn2 -- Controlled Voltage Source3/LConn1
  Motor2/LConn1 -- Controlled Voltage Source5/RConn1
  Motor1/LConn1 -- Controlled Voltage Source3/RConn1
  Motor2/LConn2 -- Controlled Voltage Source5/LConn1
  Motor1/LConn3 -- Controlled Voltage Source4/RConn1
  Motor2/LConn3 -- Controlled Voltage Source6/RConn1
